simulink model "sim2"  (R2024a)
settings: Solver=FixedStepAuto  StartTime=0.0  StopTime=60.0  FixedStep=1e-4  RelTol=1e-3
libraries: simulink x1
settings Model: Creator=alexe  LastModifiedBy=alexe

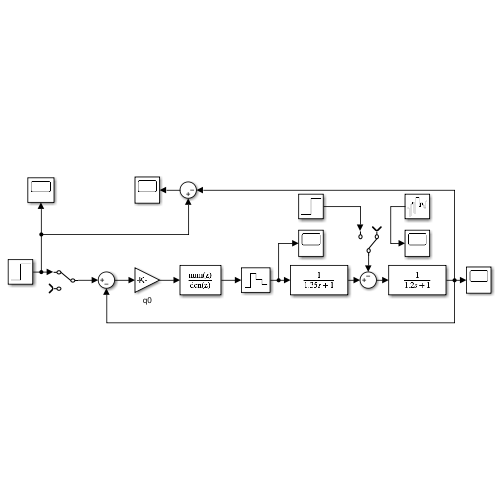
[thumbnail: Simulink's stored preview of the top-level diagram]
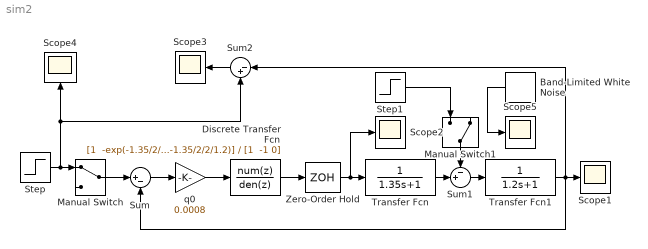
== system sim2 ==
  Band-Limited White Noise : simulink/Sources/Band-Limited White Noise  Cov=[0.01]  Ts=0.1  seed=[23341]
  Discrete Transfer Fcn : DiscreteTransferFcn  Numerator="[1  -exp(-1.35/2/2/1.35)-exp(-1.35/2/2/1.2) exp(-1.35/2/2/1.35)*exp(-1.35/2/2/1.2)]"  Denominator="[1  -1 0]"
  Manual Switch : ManualSwitch
  Manual Switch1 : ManualSwitch  CurrentSetting=0
  Scope{1..5} (5 alike) : Scope
  Step : Step  SampleTime=0
  Step1 : Step  Time=10  Before=-1  SampleTime=0
  Sum : Sum  Inputs=|+-
  Sum1 : Sum  Inputs=-+|
  Sum2 : Sum  Inputs=|-+
  Transfer Fcn : TransferFcn  Denominator=[1.35 1]
  Transfer Fcn1 : TransferFcn  Denominator=[1.2 1]
  Zero-Order Hold : ZeroOrderHold  SampleTime=1.35/4
  q0 : Gain  Gain=0.0008
  wires:
  Step/1 -> Sum2/2, Scope4/1, Manual Switch/1
  Manual Switch/1 -> Sum/1
  q0/1 -> Discrete Transfer Fcn/1
  Discrete Transfer Fcn/1 -> Zero-Order Hold/1
  Zero-Order Hold/1 -> Scope2/1, Transfer Fcn/1
  Transfer Fcn/1 -> Sum1/2
  Sum1/1 -> Transfer Fcn1/1
  Transfer Fcn1/1 -> Sum2/1, Sum/2, Scope1/1
  Step1/1 -> Manual Switch1/1
  Manual Switch1/1 -> Sum1/1
  Sum/1 -> q0/1
  Sum2/1 -> Scope3/1
  Band-Limited White Noise/1 -> Scope5/1
